simulink model "LQG_sim"  (Simulink 7.5)
settings: Solver=ode45  StartTime=0.0  StopTime=40  RelTol=1e-3
InitFcn:
  | start_lqg
values from neighbouring files (symbols this model uses):
  A = [-0.1778 0 0 0 0 -9.7807 -9.7807 0 0 0 0 ... (first row only)    [start_h2.m]    (also in start_hinf.m; start_lqg.m)
  B = [zeros(6,4) ... (first row only)    [start_h2.m]    (also in start_hinf.m; start_lqg.m)
  C = [eye(6,11); zeros(2,8) [1 0 0; 0 1 0]]    [start_h2.m]    (also in start_hinf.m; start_lqg.m)
  E = [A(:,1),A(:,2),A(:,9)]    [start_h2.m]    (also in start_hinf.m; start_lqg.m)
  K = -(Q*C1'+Ecap*D1')/(D1*D1')    [start_h2.m]    (also in start_hinf.m = -(Q*C1'+Ecap*D1')*inv((D1*D1')))
  x0 = [1 0 0 0 0 -0.1 0 0 0 0 0]'    [start_h2.m]    (also in start_hinf.m; start_lqg.m)
undefined symbols (not defined in the file or in its folder): L
settings Model: Creator=Prasad  LastModifiedBy=Prasad

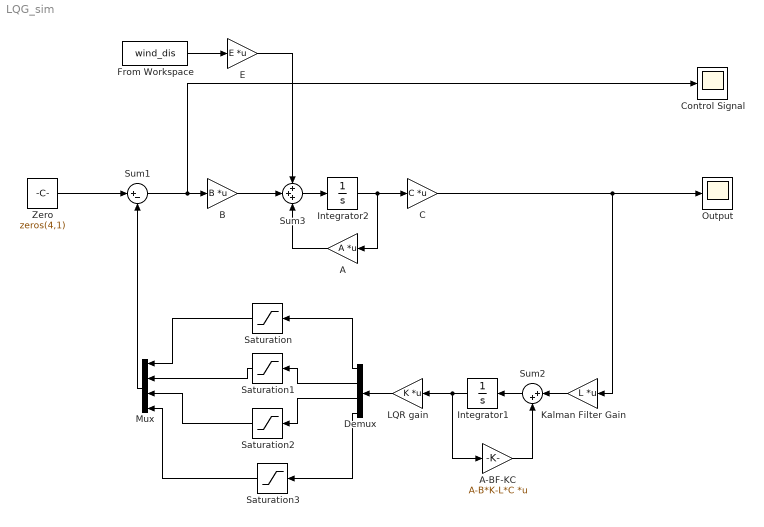
== system LQG_sim ==
  A : Gain  Gain=A  Multiplication=Matrix(K*u)  ParameterDataType=fixdt(1, 16)  ParameterScaling=2^0  OutDataType=fixdt(1, 16)  OutScaling=2^0
  A-BF-KC : Gain  Gain=A-B*K-L*C  Multiplication=Matrix(K*u)  ParameterDataType=fixdt(1, 16)  ParameterScaling=2^0  OutDataType=fixdt(1, 16)  OutScaling=2^0
  B : Gain  Gain=B  Multiplication=Matrix(K*u)  ParameterDataType=fixdt(1, 16)  ParameterScaling=2^0  OutDataType=fixdt(1, 16)  OutScaling=2^0
  C : Gain  Gain=C  Multiplication=Matrix(K*u)  ParameterDataType=fixdt(1, 16)  ParameterScaling=2^0  OutDataType=fixdt(1, 16)  OutScaling=2^0
  Control Signal : Scope
      settings: TimeRange=10  YMin=-0.4  YMax=1.2
  Demux : Demux
  E : Gain  Gain=E  Multiplication=Matrix(K*u)  ParameterDataType=fixdt(1, 16)  ParameterScaling=2^0  OutDataType=fixdt(1, 16)  OutScaling=2^0
  From Workspace : FromWorkspace  VariableName=wind_dis  SampleTime=0  OutputAfterFinalValue=Holding final value
  Integrator1 : Integrator
  Integrator2 : Integrator  InitialCondition=x0
  Kalman Filter Gain : Gain  Gain=L  Multiplication=Matrix(K*u)  ParameterDataType=fixdt(1, 16)  ParameterScaling=2^0  OutDataType=fixdt(1, 16)  OutScaling=2^0
  LQR gain : Gain  Gain=K  Multiplication=Matrix(K*u)  ParameterDataType=fixdt(1, 16)  ParameterScaling=2^0  OutDataType=fixdt(1, 16)  OutScaling=2^0
  Mux : Mux
  Output : Scope
      settings: TimeRange=10  YMin=-0.4  YMax=1.2
  Saturation : Saturate  UpperLimit=0.35  LowerLimit=-0.35  OutDataType=fixdt(1, 16)  OutScaling=2^0
  Saturation1 : Saturate  UpperLimit=0.35  LowerLimit=-0.35  OutDataType=fixdt(1, 16)  OutScaling=2^0
  Saturation2 : Saturate  UpperLimit=0.12  LowerLimit=-0.12  OutDataType=fixdt(1, 16)  OutScaling=2^0
  Saturation3 : Saturate  UpperLimit=0.4  LowerLimit=-0.4  OutDataType=fixdt(1, 16)  OutScaling=2^0
  Sum1 : Sum  Inputs=|+-  OutDataType=fixdt(1, 16)  OutScaling=2^0
  Sum2 : Sum  Inputs=|++  OutDataType=fixdt(1, 16)  OutScaling=2^0
  Sum3 : Sum  Inputs=+++  OutDataType=fixdt(1, 16)  OutScaling=2^0
  Zero : Constant  Value=zeros(4,1)  OutDataType=fixdt(1, 16)  OutScaling=2^0
  wires:
  Sum1/1 -> B/1, Control Signal/1
  Integrator1/1 -> LQR gain/1, A-BF-KC/1
  Sum2/1 -> Integrator1/1
  A-BF-KC/1 -> Sum2/2
  Kalman Filter Gain/1 -> Sum2/1
  C/1 -> Kalman Filter Gain/1, Output/1
  Demux/1 -> Saturation/1
  Demux/2 -> Saturation1/1
  Demux/3 -> Saturation2/1
  Demux/4 -> Saturation3/1
  Saturation/1 -> Mux/1
  Saturation1/1 -> Mux/2
  Saturation2/1 -> Mux/3
  Saturation3/1 -> Mux/4
  LQR gain/1 -> Demux/1
  Mux/1 -> Sum1/2
  Sum3/1 -> Integrator2/1
  Integrator2/1 -> C/1, A/1
  E/1 -> Sum3/1
  A/1 -> Sum3/3
  From Workspace/1 -> E/1
  B/1 -> Sum3/2
  Zero/1 -> Sum1/1
